simulink model "mpc_lateral_control"  (R2022a)
settings: Solver=ode3  StartTime=0.0  StopTime=inf  FixedStep=0.005  RelTol=1e-3
undefined symbols (not defined in the file): Angular, Linear
libraries: robotlib x5, mpclib x1, robotcorelib x1
settings Model: Creator=Ronak Jain  LastModifiedBy=Ronak Jain
settings OptimizationCC: EnhancedBackFolding=on  PassReuseOutputArgsAs=Individual arguments  LifeSpan=inf  MaxStackSize=64  OptimizeBlockOrder=speed  DifferentSizesBufferReuse=on  OptimizationCustomize=off  EfficientTunableParamExpr=on
settings DebuggingCC: ParameterTunabilityLossMsg=error  BusObjectLabelMismatch=error
settings HardwareCC: ProdBitPerPointer=32  ProdBitPerSizeT=32  ProdBitPerPtrDiffT=32  ProdLargestAtomicFloat=None  ProdIntDivRoundTo=Undefined  ProdEndianess=Unspecified  ProdWordSize=32  ProdHWDeviceType=Generic->Unspecified (assume 32-bit Generic)  TargetBitPerPointer=64  TargetBitPerSizeT=64  TargetBitPerPtrDiffT=64  TargetLongLongMode=on  TargetIntDivRoundTo=Zero  TargetEndianess=LittleEndian  TargetWordSize=64  TargetHWDeviceType=MATLAB Host  ProdEqTarget=off
settings RTWCC: SystemTargetFile=ert.tlc  HardwareBoard=Robot Operating System (ROS)  TLCOptions="-aInlineSetEventsForThisBaseRateFcn=TLC_FALSE -aSuppressMultiTaskScheduler=TLC_FALSE  -aRateBasedStepFcn=0"  TemplateMakefile=ert_default_tmf  Toolchain=Catkin  TargetLang=C++
settings CodeAppCC: ForceParamTrailComments=on  IgnoreCustomStorageClasses=off  OperatorAnnotations=on  SimulinkDataObjDesc=on  SFDataObjDesc=on  InsertBlockDesc=on
settings ERTTargetCC: CodeInterfacePackaging=Reusable function  SupportContinuousTime=on  SupportVariableSizeSignals=on  ModelStepFunctionPrototypeControlCompliant=off  GenerateAllocFcn=on  MultiInstanceErrorCode=None  RootIOFormat=Part of model data structure

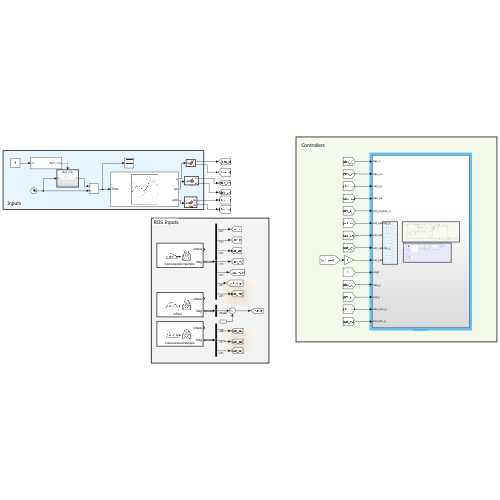
[thumbnail: Simulink's stored preview of the top-level diagram]
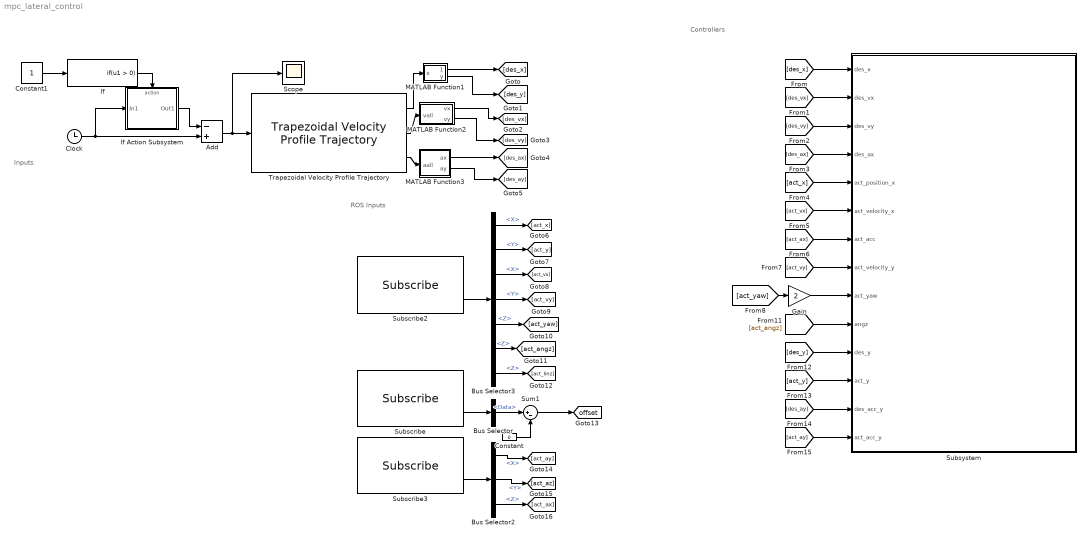
== system mpc_lateral_control ==
  note: Inputs
  note: ROS Inputs
  note: Controllers
  Add : Sum  Inputs=-+
  Bus Selector : BusSelector  OutputSignals=Data
  Bus Selector2 : BusSelector  OutputSignals=LinearAcceleration.X,LinearAcceleration.Y,LinearAcceleration.Z
  Bus Selector3 : BusSelector  OutputSignals=Pose.Pose.Position.X,Pose.Pose.Position.Y,Twist.Twist.Linear.X,Twist.Twist.Linear.Y,Pose.Pose.Orientation.Z,Twist.Twist.Angular.Z,Twist.Twist.Linear.Z
  Clock : Clock
  Constant : Constant  Value=0
  Constant1 : Constant  SampleTime=-1
  Gain : Gain  Gain=2
  If : If  ShowElse=off
  If Action Subsystem : Subsystem  TreatAsAtomicUnit=on
  MATLAB Function1 : MATLAB Function  TreatAsAtomicUnit=on
  MATLAB Function2 : MATLAB Function  TreatAsAtomicUnit=on
  MATLAB Function3 : MATLAB Function  TreatAsAtomicUnit=on
  Scope : Scope
  Subscribe : robotlib/Subscribe  topicSource=Select from ROS network  topic=/offset  messageType=std_msgs/Float32  SampleTime=-1  legacyBusStruct=off  messageQueueLength=1
  Subscribe2 : robotlib/Subscribe  topicSource=Select from ROS network  topic=/camera/odom/sample  messageType=nav_msgs/Odometry  SampleTime=-1  legacyBusStruct=off  messageQueueLength=1
  Subscribe3 : robotlib/Subscribe  topicSource=Select from ROS network  topic=/camera/accel/sample  messageType=sensor_msgs/Imu  SampleTime=-1  legacyBusStruct=off  messageQueueLength=1
  Subsystem : Subsystem
  Sum1 : Sum  Inputs=|+-
  Trapezoidal Velocity Profile Trajectory : robotcorelib/Trapezoidal Velocity Profile Trajectory  WaypointSource=Internal  Waypoints=[0,2.5*3;0,0]  NumParams=2  Parameter1=Acceleration Time  Parameter2=End Time  ParameterSource=Internal  PeakVelocity=[ 2; 2 ]  Acceleration=[ 1; 2 ]  EndTime=[ 35*3;35*3]  AccelTime=[ 10; 10 ]  SimulateUsing=Interpreted execution
      settings: SourceProductBaseCode=RO,NV,RR,UV
  tag scope: offset=global
  wires:
  Subscribe3/2 -> Bus Selector2/1
  Trapezoidal Velocity Profile Trajectory/1 -> MATLAB Function1/1(x)
  If Action Subsystem/1(Out1) -> Add/1
  Subscribe2/2 -> Bus Selector3/1
  Subscribe/2 -> Bus Selector/1
  If/1 -> If Action Subsystem/Action
  Trapezoidal Velocity Profile Trajectory/2 -> MATLAB Function2/1(vall)
  Trapezoidal Velocity Profile Trajectory/3 -> MATLAB Function3/1(aall)
  Constant1/1 -> If/1
  Clock/1 -> Add/2, If Action Subsystem/1(In1)
  Add/1 -> Scope/1, Trapezoidal Velocity Profile Trajectory/1
  MATLAB Function1/1(x1) -> [des_x]
  MATLAB Function1/2(y) -> [des_y]
  MATLAB Function2/1(vx) -> [des_vx]
  MATLAB Function2/2(vy) -> [des_vy]
  MATLAB Function3/1(ax) -> [des_ax]
  MATLAB Function3/2(ay) -> [des_ay]
  Bus Selector3/1 -> [act_x]  "<X>"
  Bus Selector3/2 -> [act_y]  "<Y>"
  Bus Selector3/3 -> [act_vx]  "<X>"
  Bus Selector3/4 -> [act_vy]  "<Y>"
  Bus Selector3/5 -> [act_yaw]  "<Z>"
  Bus Selector3/6 -> [act_angz]  "<Z>"
  Bus Selector3/7 -> [act_linz]  "<Z>"
  Bus Selector2/1 -> [act_ay]  "<X>"
  Bus Selector2/2 -> [act_az]  "<Y>"
  Bus Selector2/3 -> [act_ax]  "<Z>"
  [des_x] -> Subsystem/1(des_x)
  [des_vx] -> Subsystem/2(des_vx)
  [des_vy] -> Subsystem/3(des_vy)
  [des_ax] -> Subsystem/4(des_ax)
  [act_x] -> Subsystem/5(act_position_x)
  [act_vx] -> Subsystem/6(act_velocity_x)
  [act_ax] -> Subsystem/7(act_acc)
  [act_vy] -> Subsystem/8(act_velocity_y)
  [act_yaw] -> Gain/1
  [act_angz] -> Subsystem/10(angz)
  [des_y] -> Subsystem/11(des_y)
  [act_y] -> Subsystem/12(act_y)
  [des_ay] -> Subsystem/13(des_acc_y)
  [act_ay] -> Subsystem/14(act_acc_y)
  Gain/1 -> Subsystem/9(act_yaw)
  Bus Selector/1 -> Sum1/1  "<Data>"
  Sum1/1 -> [offset]
  Constant/1 -> Sum1/2

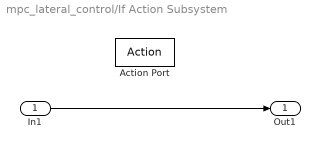
== system mpc_lateral_control/If Action Subsystem ==
  In1 : Inport
  Action Port : ActionPort  PropagateVarSize=During execution  ActionPortLabel=if(u1 > 0)
  Out1 : Outport
  wires:
  In1/1 -> Out1/1

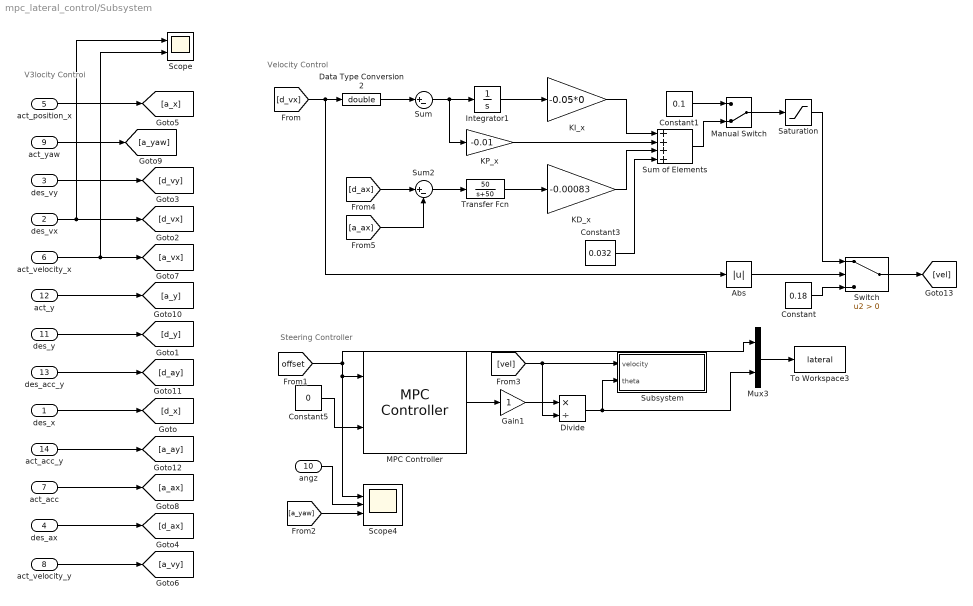
== system mpc_lateral_control/Subsystem ==
  note: Velocity Control
  note: Steering Controller
  note: V3locity Controi
  des_x : Inport
  des_vx : Inport  Port=2
  des_vy : Inport  Port=3
  des_ax : Inport  Port=4
  act_position_x : Inport  Port=5
  act_velocity_x : Inport  Port=6
  act_acc : Inport  Port=7
  act_velocity_y : Inport  Port=8
  act_yaw : Inport  Port=9
  angz : Inport  Port=10
  des_y : Inport  Port=11
  act_y : Inport  Port=12
  des_acc_y : Inport  Port=13
  act_acc_y : Inport  Port=14
  Abs : Abs  SaturateOnIntegerOverflow=off
  Constant : Constant  Value=0.18
  Constant1 : Constant  Value=0.1
  Constant3 : Constant  Value=0.032
  Constant5 : Constant  Value=0
  Data Type Conversion2 : DataTypeConversion  OutDataTypeStr=double  SaturateOnIntegerOverflow=off  RndMeth=Floor
  Divide : Product  Inputs=*/
  Gain1 : Gain
  Integrator1 : Integrator
  KD_x : Gain  Gain=-0.00083
  KI_x : Gain  Gain=-0.05*0
  KP_x : Gain  Gain=-0.01
  MPC Controller : mpclib/MPC Controller  SCDEnableBlockLinearizationSpecification=on  mpcobj=mpc1  is_multiple=0  enable_value=0  return_u0=off  updateMPCinCallerWorkspace=on  md_inport=off  mv_inport=off  uref_inport=off  return_cost=off  return_mvseq=off  return_qpstatus=off  return_xseq=off  return_state=off  return_ovseq=off  state_inport=off  umin_inport=off  umax_inport=off  ymin_inport=off  ymax_inport=off  cc_inport=off  ywt_inport=off  uwt_inport=off  duwt_inport=off  rhoeps_inport=off  pm_inport=off  MaximumP=10  HorizonChoice=FixedHorizon  n_ts=0.01  n_p=42  n_mv=1  n_md=1  n_ud=0  n_mo=1  n_uo=0  BlockDataType=double  SampleTimeInherited=off  switch_inport=off
  Manual Switch : ManualSwitch  CurrentSetting=0
  Mux3 : Mux  Inputs=2
  Saturation : Saturate  LowerLimit=-0.2
  Scope : Scope  NumInputPorts=2
  Scope4 : Scope  NumInputPorts=5
  Subsystem : Subsystem
  Sum : Sum  Inputs=|+-
  Sum of Elements : Sum  Inputs=++++
  Sum2 : Sum  Inputs=|+-
  Switch : Switch  Criteria=u2 > Threshold  SaturateOnIntegerOverflow=off  InputSameDT=off
  To Workspace3 : ToWorkspace  VariableName=lateral  SaveFormat=Timeseries  SampleTime=-1
  Transfer Fcn : TransferFcn  Numerator=[50]  Denominator=[1 50]
  wires:
  KD_x/1 -> Sum of Elements/3
  Mux3/1 -> To Workspace3/1
  Abs/1 -> Switch/2
  des_vx/1 -> Scope/1, [d_vx]
  des_vy/1 -> [d_vy]
  Constant/1 -> Switch/3
  MPC Controller/1 -> Gain1/1
  Transfer Fcn/1 -> KD_x/1
  Manual Switch/1 -> Saturation/1
  Switch/1 -> [vel]
  angz/1 -> Scope4/3
  Sum of Elements/1 -> Manual Switch/2
  Saturation/1 -> Switch/1
  Constant1/1 -> Manual Switch/1
  Constant3/1 -> Sum of Elements/4
  [offset] -> Scope4/2, MPC Controller/1, Mux3/1
  [a_ax] -> Sum2/2
  [d_ax] -> Sum2/1
  Sum2/1 -> Transfer Fcn/1
  KI_x/1 -> Sum of Elements/1
  Integrator1/1 -> KI_x/1
  act_velocity_y/1 -> [a_vy]
  act_yaw/1 -> [a_yaw]
  KP_x/1 -> Sum of Elements/2
  Data Type Conversion2/1 -> Sum/1
  Sum/1 -> KP_x/1, Integrator1/1
  Divide/1 -> Mux3/2, Subsystem/2(theta)
  des_x/1 -> [d_x]
  [d_vx] -> Data Type Conversion2/1, Abs/1
  des_acc_y/1 -> [d_ay]
  act_acc_y/1 -> [a_ay]
  des_y/1 -> [d_y]
  act_y/1 -> [a_y]
  act_velocity_x/1 -> Scope/2, [a_vx]
  act_acc/1 -> [a_ax]
  des_ax/1 -> [d_ax]
  act_position_x/1 -> [a_x]
  Gain1/1 -> Divide/1
  Constant5/1 -> MPC Controller/2
  [a_yaw] -> Scope4/4
  [vel] -> Divide/2, Subsystem/1(velocity)

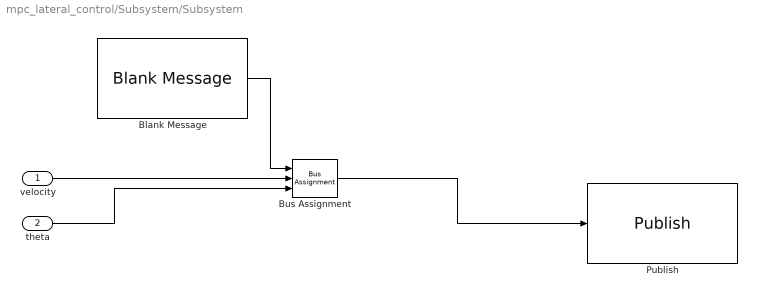
== system mpc_lateral_control/Subsystem/Subsystem ==
  velocity : Inport
  theta : Inport  Port=2
  Blank Message : robotlib/Blank Message  messageClass=Message  entityType=geometry_msgs/Twist  messageType=geometry_msgs/Twist  SampleTime=-1  legacyBusStruct=off
  Bus Assignment : BusAssignment  AssignedSignals=Linear.X,Angular.Z
  Publish : robotlib/Publish  topicSource=Specify your own  topic=/move_velocity  messageType=geometry_msgs/Twist  legacyBusStruct=off  messageQueueLength=1
  wires:
  theta/1 -> Bus Assignment/3
  Blank Message/1 -> Bus Assignment/1
  velocity/1 -> Bus Assignment/2
  Bus Assignment/1 -> Publish/1

== matlab function mpc_lateral_control/MATLAB Function2 ==
  data: vall input; vx output; vy output
function [vx,vy] = fcn(vall)
vx = vall(1,:);
vy = vall(2,:);

== matlab function mpc_lateral_control/MATLAB Function3 ==
  data: aall input; ax output; ay output
function [ax,ay]  = fcn(aall)
ax = aall(1,:);
ay = aall(2,:);
end

== matlab function mpc_lateral_control/MATLAB Function1 ==
  data: x1 output; x input; y output
function [x1,y] = fcn(x)

x1 = x(1,:);
y  = x(2,:);

end
